simulink model "Sim_MIL"  (R2026a)
settings: Solver=VariableStepAuto  StopTime=540  FixedStep=0.001  RelTol=1e-4
settings Model: Creator=tom  LastModifiedBy=Dante P
settings DebuggingCC: SignalInfNanChecking=warning

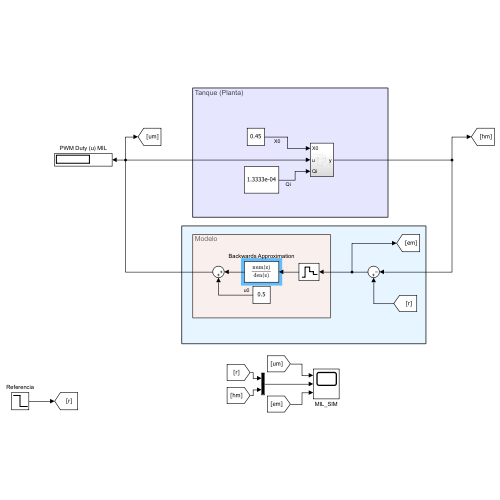
[thumbnail: Simulink's stored preview of the top-level diagram]
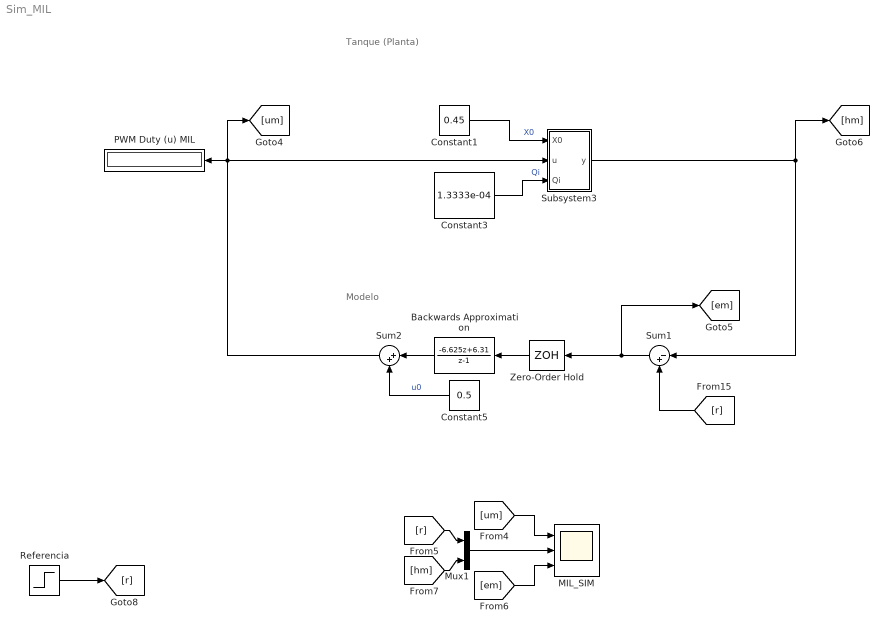
== system Sim_MIL ==
  note: Tanque (Planta)
  note: Modelo
  Backwards Approximation : DiscreteTransferFcn  Numerator=[-6.625, 6.31]  Denominator=[1, -1]  SampleTime=1  a0EqualsOne=on  StateName=C_for
  Constant1 : Constant  Value=0.45
  Constant3 : Constant  Value=1.3333e-04
  Constant5 : Constant  Value=0.5
  MIL_SIM : Scope  NumInputPorts=3
      settings: TimeSpan=500  ActiveDisplayYMinimum=0.40489468022471242  ActiveDisplayYMaximum=0.92452625415798884  YLabel=PWM Duty, u  DataLoggingVariableName=ScopeData2
  Mux1 : Mux  Inputs=2
  PWM Duty (u) MIL : Display
      settings: Format=decimal (Stored Integer)
  Referencia : Step  Time=10  InitialValue=0.45  FinalValue=0.4  SampleTime=0
  Subsystem3 : Subsystem
  Sum1 : Sum  Inputs=|-+
  Sum2 : Sum  Inputs=|++
  Zero-Order Hold : ZeroOrderHold
  wires:
  Subsystem3/1(y) -> [hm], Sum1/1
  [em] -> MIL_SIM/3
  [um] -> MIL_SIM/1
  [r] -> Mux1/1
  Constant1/1 -> Subsystem3/1(X0)  "X0"
  [hm] -> Mux1/2
  Constant3/1 -> Subsystem3/3(Qi)  "Qi"
  Constant5/1 -> Sum2/2  "u0"
  Sum2/1 -> [um], PWM Duty (u) MIL/1, Subsystem3/2(u)
  Sum1/1 -> Zero-Order Hold/1, [em]
  Zero-Order Hold/1 -> Backwards Approximation/1
  Referencia/1 -> [r]
  [r] -> Sum1/2
  Backwards Approximation/1 -> Sum2/1
  Mux1/1 -> MIL_SIM/2

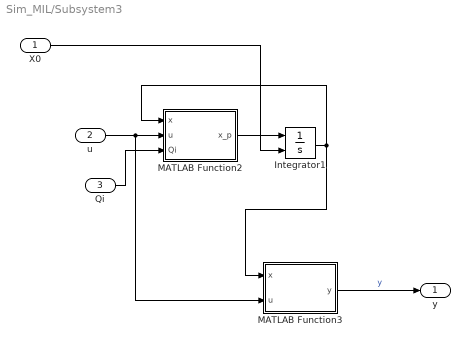
== system Sim_MIL/Subsystem3 ==
  X0 : Inport
  u : Inport  Port=2
  Qi : Inport  Port=3
  Integrator1 : Integrator  InitialConditionSource=external
  MATLAB Function2 : MATLAB Function  TreatAsAtomicUnit=on
  MATLAB Function3 : MATLAB Function  TreatAsAtomicUnit=on
  y : Outport
  wires:
  X0/1 -> Integrator1/2
  Integrator1/1 -> MATLAB Function3/1(x), MATLAB Function2/1(x)
  u/1 -> MATLAB Function3/2(u), MATLAB Function2/2(u)
  MATLAB Function2/1(x_p) -> Integrator1/1
  MATLAB Function3/1(y) -> y/1  "y"
  Qi/1 -> MATLAB Function2/3(Qi)

== matlab function Sim_MIL/Subsystem3/MATLAB Function3 ==
  data: x input; u input; y output
function y = g(x, u)
    y = x;

== matlab function Sim_MIL/Subsystem3/MATLAB Function2 ==
  data: x input size=1; u input size=1; x_p output size=1; Qi input
function x_p = f(x, u, Qi)
    d = 0.01065;
    L1 = 0.1;
    L2 = 0.4;
    L = 0.9;
    g = 9.8;
    x_p = (-sqrt(abs(2*g*x))*d^2/4*u*pi + Qi)/(L1+(L2-L1)*x/L)^2;
